simulink model "OMAP_ver_MIL10"  (R2018b)
settings: Solver=FixedStepDiscrete  StartTime=0.0  StopTime=10.0  FixedStep=0.01  RelTol=1e-3
undefined symbols (not defined in the file or in its folder): OMAP_Switch_EMS, OMAP_Switch_EPS, OMAP_Switch_ESC, OMAP_Switch_IC, OMAP_Switch_OTHER, TH_HMIClb_tiDgrdIconWarnHiDurT_C, TH_HMIClb_tiDgrdIconWarnLoDurT_C, TH_HMIClb_tiDgrdVocWarnDurT_C, TH_HMIClb_tiHndOffTxtWarnT_C, TH_HMIClb_tiHndOffVocWarnT_C, TH_HMIClb_tiSWALimFlgDetT_C, TH_HMIClb_tiTxtLimT_C
libraries: simulink x118
(part 9 of 9)

== matlab function OMAP_ver_MIL10/OMAP_Module/ICA_Direct_G59/ICA_Define/Subsystem1/Subsystem/MATLAB Function ==
  data: TH_Mode input; LC_Scene input; TSR_Version_Only_Sign_Type output; stLCRMode input
function TSR_Version_Only_Sign_Type = fcn(TH_Mode,LC_Scene,stLCRMode)
Left_Turn=uint16(16);
Right_Turn=uint16(15);
No_Turn=uint16(0);
ZERO=uint16(0);
ONE=uint16(1);
TWO=uint16(2);
THREE=uint16(3);
if(TH_Mode~=uint16(4))
    if(stLCRMode==TWO)
        TSR_Version_Only_Sign_Type=Left_Turn;
    elseif(stLCRMode==THREE)
        TSR_Version_Only_Sign_Type=Right_Turn;   
    else
        TSR_Version_Only_Sign_Type=No_Turn;   
    end
else
    if(LC_Scene==ONE)  %Left
       TSR_Version_Only_Sign_Type=Left_Turn;
    elseif(LC_Scene==TWO)
        TSR_Version_Only_Sign_Type=Right_Turn;   
    else
        TSR_Version_Only_Sign_Type=No_Turn;  
    end
end
end

== stateflow chart OMAP_ver_MIL10/OMAP_Module/ACCS_Direct/ACCS_Define/Human_Machine_Interface(ACC_HMI)/Subsystem/Chart ==
  state ObjOutRange
    en:
    Value = uint8(5);
  state ObjInRange
    state Middle
      en:
      Value = uint8(2);
    state Far
      en:
      Value = uint8(4);
    state Close
      en:
      Value = uint8(1);
    (default) -> (junction 14)
    (junction 14) -> Far [order 2] : [Distance>single(80)]
    (junction 14) -> Close [order 1] : [Distance<=single(30)]
    (junction 14) -> Middle [order 3]
    Far -> Middle [order 1] : [(Distance>single(30))&&(Distance<single(77))]
    Middle -> Close [order 1] : [Distance<single(27)]
    Middle -> Far [order 2] : [Distance>single(80)]
    Close -> Middle [order 1] : [(Distance>single(30))&&(Distance<=single(80))]
    Close -> Far [order 2] : [Distance>single(80)]
    Far -> Close [order 2] : [Distance<=single(30)]
  (default) -> (junction 28)
  (junction 28) -> ObjInRange [order 1] : [(Distance>=single(0))&&(Distance<=single(150))]
  (junction 28) -> ObjOutRange [order 2]
  ObjInRange -> ObjOutRange : [(Distance<single(0))||(Distance>single(150))]
  ObjOutRange -> ObjInRange : [(Distance>=single(0))&&(Distance<=single(150))]
  data: Distance input; Value output uint8

== stateflow chart OMAP_ver_MIL10/OMAP_Module/ACCS_Direct/ACCS_Define/Human_Machine_Interface(ACC_HMI)/Text_PopUp/ Radar_Blocked/Chart ==
  state StandBy
    en:
    Value = data;
  state Trigger
    en:
    Value = data;
  (default) -> StandBy
  StandBy -> Trigger : [data==1]
  Trigger -> StandBy : [after(3,sec)]
  data: data input; Value output boolean

== stateflow chart OMAP_ver_MIL10/OMAP_Module/ACCS_Direct/ACCS_Define/Human_Machine_Interface(ACC_HMI)/Text_PopUp/ACC_Activation_Unsatisfied/Chart ==
  state StandBy
    en:
    Value = data;
  state Trigger
    en:
    Value = data;
  (default) -> StandBy
  StandBy -> Trigger : [data==1]
  Trigger -> StandBy : [after(3,sec)]
  data: data input; Value output boolean

== stateflow chart OMAP_ver_MIL10/OMAP_Module/ACCS_Direct/ACCS_Define/Human_Machine_Interface(ACC_HMI)/Text_PopUp/ACC_Active/Chart ==
  state StandBy
    en:
    Value = data;
  state Trigger
    en:
    Value = data;
  (default) -> StandBy
  StandBy -> Trigger : [data==1]
  Trigger -> StandBy : [after(3,sec)]
  data: data input; Value output boolean

== stateflow chart OMAP_ver_MIL10/OMAP_Module/ACCS_Direct/ACCS_Define/Human_Machine_Interface(ACC_HMI)/Text_PopUp/ACC_Canceled/Chart ==
  state StandBy
    en:
    Value = data;
  state Trigger
    en:
    Value = data;
  (default) -> StandBy
  StandBy -> Trigger : [data==1]
  Trigger -> StandBy : [after(3,sec)]
  data: data input; Value output boolean

== stateflow chart OMAP_ver_MIL10/OMAP_Module/ACCS_Direct/ACCS_Define/Human_Machine_Interface(ACC_HMI)/Text_PopUp/ACC_Fault/Chart ==
  state StandBy
    en:
    Value = data;
  state Trigger
    en:
    Value = data;
  (default) -> StandBy
  StandBy -> Trigger : [data==1]
  Trigger -> StandBy : [after(3,sec)]
  data: data input; Value output boolean

== stateflow chart OMAP_ver_MIL10/OMAP_Module/ACCS_Direct/ACCS_Define/Human_Machine_Interface(ACC_HMI)/Text_PopUp/ACC_OFF/Chart ==
  state StandBy
    en:
    Value = data;
  state Trigger
    en:
    Value = data;
  (default) -> StandBy
  StandBy -> Trigger : [(data==1)&&(data1==0)]
  Trigger -> StandBy : [after(3,sec)]
  data: data input; Value output boolean; data1 input

== stateflow chart OMAP_ver_MIL10/OMAP_Module/ACCS_Direct/ACCS_Define/Human_Machine_Interface(ACC_HMI)/Text_PopUp/ACC_ON/Chart ==
  state StandBy
    en:
    Value = data;
  state Trigger
    en:
    Value = data;
  state Trigger1
    en:
    Value = data2;
  (default) -> StandBy
  StandBy -> Trigger [order 1] : [data==1]
  Trigger -> StandBy : [after(6,sec)||(data1==1)]
  Trigger1 -> StandBy : [after(6,sec)||(data1==1)]
  StandBy -> Trigger1 [order 2] : [data2==1]
  data: data input; Value output boolean; data1 input; data2 input

== stateflow chart OMAP_ver_MIL10/OMAP_Module/ACCS_Direct/ACCS_Define/Human_Machine_Interface(ACC_HMI)/Text_PopUp/Please_Take_Over_the_Car/Chart1 ==
  state StandBy
    en:
    Value = uint8(0);
  state Trigger
    en:
    Value = uint8(1);
  (default) -> StandBy
  StandBy -> Trigger : [IN==1]
  Trigger -> StandBy : [OUT==1]
  data: IN input boolean; OUT input boolean; Value output uint8

== stateflow chart OMAP_ver_MIL10/OMAP_Module/ACCS_Direct/ACCS_Define/Human_Machine_Interface(ACC_HMI)/Text_PopUp/Please_Take_Over_the_Car_immediataly/Chart1 ==
  state StandBy1
    en:
    Value = uint8(0);
  state Trigger
    en:
    Value = uint8(1);
  state StandBy
    en:
    Value = uint8(0);
  (default) -> StandBy
  StandBy -> StandBy1 : [(ESC_DecTar>-5)&&(ESC_DecTar<-3)]
  StandBy1 -> Trigger [order 2] : [after(4,sec)]
  StandBy1 -> StandBy [order 1] : [ESC_DecTar>-3]
  Trigger -> StandBy : [ESC_DecTar>-3]
  data: ESC_DecTar input single; Value output uint8; BRAKE_RELEASED_FAILSAFE input
